simulink model "ofdm_demo"  (Simulink 7.6)
settings: Solver=ode45  StartTime=0.0  StopTime=inf  RelTol=1e-3
libraries: dspmtrx3 x6, commchan3 x2, commdigbbndpm3 x2, dspxfrm3 x2, commrandsrc2 x1, commsink2 x1
settings Model: Creator=Administrator  LastModifiedBy=Administrator

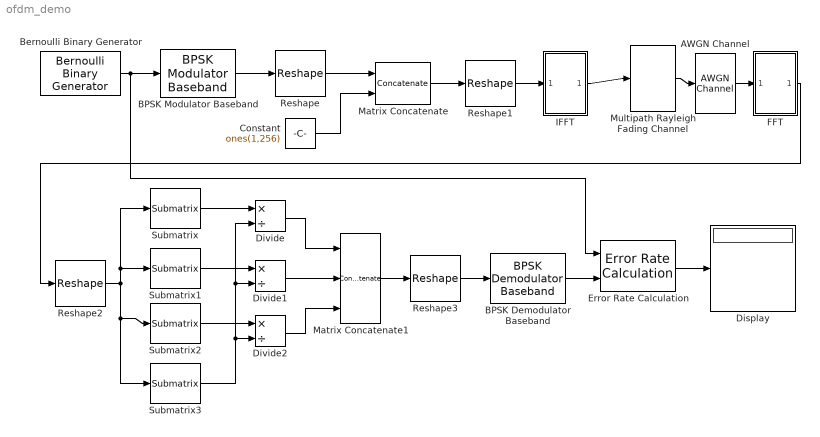
== system ofdm_demo ==
  AWGN Channel : commchan3/AWGN Channel  SystemSampleTime=-1  InputProcessing=Columns as channels (frame based)  seed=67  noiseMode="Signal to noise ratio  (Eb/No)"  EbNodB=10  EsNodB=10  SNRdB=10  bitsPerSym=1  Ps=1  Tsym=1e-6  variance=1
  BPSK Demodulator Baseband : commdigbbndpm3/BPSK Demodulator Baseband  DialogController=commDDGCreate  DialogControllerArgs=DataTag1  Ph=0  DecType=Hard decision  VarSource=Dialog  Variance=1  outDtype=Inherit via internal rule  derotateFactorWordLen=16
  BPSK Modulator Baseband : commdigbbndpm3/BPSK Modulator Baseband  DialogController=commDDGCreate  DialogControllerArgs=DataTag2  SystemSampleTime=-1  Ph=0  outDtype=double  outWordLen=16  outUDDataType=sfix(16)  outFracLenMode=Best precision  outFracLen=15
  Bernoulli Binary Generator : commrandsrc2/Bernoulli Binary Generator  DialogController=commDDGCreate  DialogControllerArgs=DataTag3  SystemSampleTime=-1  P=0.5  seed=61  Ts=1e-6  frameBased=on  sampPerFrame=768  orient=off  outDataType=double
  Constant : Constant  Value=ones(1,256)  VectorParams1D=off
      settings: SamplingMode=Frame based
  Display : Display
  Divide : Product  Inputs=*/
  Divide1 : Product  Inputs=*/
  Divide2 : Product  Inputs=*/
  Error Rate Calculation : commsink2/Error Rate Calculation  N=0  st_delay=0  cp_mode=Entire frame  subframe=[]  PMode=Port  WsName=ErrorVec  RsMode2=off  stop=off  numErr=100  maxBits=1e6
  FFT : Subsystem
  IFFT : Subsystem
  Matrix Concatenate : Concatenate  Mode=Multidimensional array
  Matrix Concatenate1 : Concatenate  NumInputs=3  Mode=Multidimensional array
  Multipath Rayleigh Fading Channel : commchan3/Multipath Rayleigh Fading Channel  SystemSampleTime=-1  maxDopplerShift=40  spectrumType=Jakes  sigmaGaussian=1/sqrt(2)  coeffRounded=[1 -1.72 0.785]  freqMinMaxRJakes=[0 1]  freqMinMaxAJakes=[0 1]  sigmaGaussian1=1/sqrt(2)  sigmaGaussian2=1/sqrt(2)  centerFreqGaussian1=0.0  centerFreqGaussian2=0.0  gainGaussian1=0.5  gainGaussian2=0.5  coeffBell=9  dopplerSpectrum=doppler.jakes  pathDelays=[0 2e-6]  avgPathGaindB=[0 -3]  normalizePathGains=on  seed=73  enableProbe=0  openVisAtStart=off  outPathGains=off  outDelay=off
  Reshape : Reshape  OutputDimensionality=Customize  OutputDimensions=[3,256]
  Reshape1 : Reshape  OutputDimensionality=Customize  OutputDimensions=[1024,1]
  Reshape2 : Reshape  OutputDimensionality=Customize  OutputDimensions=[4,256]
  Reshape3 : Reshape  OutputDimensionality=Customize  OutputDimensions=[768,1]
  Submatrix : dspmtrx3/Submatrix  RowSpan=Range of rows  RowStartMode=Index  RowStartIndex=1  RowEndMode=Index  RowEndIndex=1  ColSpan=Range of columns  ColStartMode=First  ColStartIndex=1  ColEndMode=Last  ColEndIndex=1
  Submatrix1 : dspmtrx3/Submatrix  RowSpan=Range of rows  RowStartMode=Index  RowStartIndex=2  RowEndMode=Index  RowEndIndex=2  ColSpan=Range of columns  ColStartMode=First  ColStartIndex=1  ColEndMode=Last  ColEndIndex=1
  Submatrix2 : dspmtrx3/Submatrix  RowSpan=Range of rows  RowStartMode=Index  RowStartIndex=3  RowEndMode=Index  RowEndIndex=3  ColSpan=Range of columns  ColStartMode=First  ColStartIndex=1  ColEndMode=Last  ColEndIndex=1
  Submatrix3 : dspmtrx3/Submatrix  RowSpan=Range of rows  RowStartMode=Index  RowStartIndex=4  RowEndMode=Index  RowEndIndex=4  ColSpan=Range of columns  ColStartMode=First  ColStartIndex=1  ColEndMode=Last  ColEndIndex=1
  wires:
  Bernoulli Binary Generator/1 -> BPSK Modulator Baseband/1, Error Rate Calculation/1
  IFFT/1(Out1) -> Multipath Rayleigh Fading Channel/1
  AWGN Channel/1 -> FFT/1(In1)
  Multipath Rayleigh Fading Channel/1 -> AWGN Channel/1
  BPSK Modulator Baseband/1 -> Reshape/1
  Reshape/1 -> Matrix Concatenate/1
  Constant/1 -> Matrix Concatenate/2
  Matrix Concatenate/1 -> Reshape1/1
  Reshape1/1 -> IFFT/1(In1)
  FFT/1(Out1) -> Reshape2/1
  Submatrix/1 -> Divide/1
  Reshape2/1 -> Submatrix/1, Submatrix1/1, Submatrix3/1, Submatrix2/1
  Submatrix1/1 -> Divide1/1
  Submatrix2/1 -> Divide2/1
  Submatrix3/1 -> Divide/2, Divide1/2, Divide2/2
  Divide/1 -> Matrix Concatenate1/1
  Divide1/1 -> Matrix Concatenate1/2
  Divide2/1 -> Matrix Concatenate1/3
  Matrix Concatenate1/1 -> Reshape3/1
  Reshape3/1 -> BPSK Demodulator Baseband/1
  BPSK Demodulator Baseband/1 -> Error Rate Calculation/2
  Error Rate Calculation/1 -> Display/1

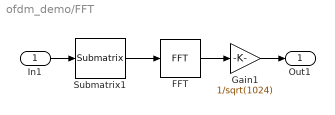
== system ofdm_demo/FFT ==
  In1 : Inport
  FFT : dspxfrm3/FFT  DialogController=dspDDGCreate  DialogControllerArgs=DataTag4  CompMethod=Table lookup  TableOpt=NEW  TableOptActive=Speed  BitRevOrder=off  InheritFFTLength=on  FFTLength=64  RowConvenienceOn=on  SkipNorm=off  firstCoeffDataTypeStr=Inherit: Same word length as input  firstCoeffLastDataTypeStr=Inherit: Same word length as input  outputMin=[]  outputMax=[]  roundingMode=Floor  overflowMode=off
  Gain1 : Gain  Gain=1/sqrt(1024)
  Submatrix1 : dspmtrx3/Submatrix  RowSpan=Range of rows  RowStartMode=Index  RowStartIndex=256+1  RowEndMode=Last  RowEndIndex=1  ColSpan=Range of columns  ColStartMode=First  ColStartIndex=1  ColEndMode=Last  ColEndIndex=1
  Out1 : Outport
  wires:
  FFT/1 -> Gain1/1
  Submatrix1/1 -> FFT/1
  Gain1/1 -> Out1/1
  In1/1 -> Submatrix1/1

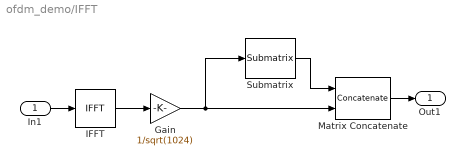
== system ofdm_demo/IFFT ==
  In1 : Inport
  Gain : Gain  Gain=1/sqrt(1024)
  IFFT : dspxfrm3/IFFT  DialogController=dspDDGCreate  DialogControllerArgs=DataTag5  CompMethod=Table lookup  TableOpt=NEW  TableOptActive=Speed  BitRevOrder=off  cs_in=off  SkipNorm=off  InheritFFTLength=on  FFTLength=64  mode=Complex  outSamplingMode=Frame based  RowConvenienceOn=on  firstCoeffDataTypeStr=Inherit: Same word length as input  firstCoeffLastDataTypeStr=Inherit: Same word length as input  outputMin=[]  outputMax=[]  roundingMode=Floor  overflowMode=off
  Matrix Concatenate : Concatenate  Mode=Multidimensional array
  Submatrix : dspmtrx3/Submatrix  RowSpan=Range of rows  RowStartMode=Index  RowStartIndex=256*3+1  RowEndMode=Last  RowEndIndex=1  ColSpan=Range of columns  ColStartMode=First  ColStartIndex=1  ColEndMode=Last  ColEndIndex=1
  Out1 : Outport
  wires:
  IFFT/1 -> Gain/1
  Gain/1 -> Submatrix/1, Matrix Concatenate/2
  Submatrix/1 -> Matrix Concatenate/1
  Matrix Concatenate/1 -> Out1/1
  In1/1 -> IFFT/1
